simulink model "flightControlSystem"  (R2022a)
settings: Solver=ode3  StartTime=0  StopTime=TFinal  FixedStep=Ts  RelTol=1e-3  EnableMultiTasking=on
model workspace (MAT data in the model file):
  CIRCLE_PTS = [19 19 19]
  ZEROS = [0 0 0 0 0 0 0 0 0 0 0 0 ... (1444 elements, 38x38)]
undefined symbols (not defined in the file): codertarget, Controller, DiscIntNeverNeededParam, Discrete, Estimator, g, gray, init, orient_ref, pos_ref, Rec, SDTV, Sensors, Time, Ts, var_acc_angle_N, var_bias_gyr_N, var_gyro_p_N, Vehicle
libraries: simulink x38, visiontextngfix x7, visionconversions x5, slpidlib x4, ctrlSharedLib x4, sharedtransform x3, visionanalysis x1, parrotlib x1
(part 3 of 3)

== system flightControlSystem/Control System/State Estimator/XY Position Estimator/EstimatorVelocity/xy velocity w//o angular velocity compensation ==
  note: Optical flow raw readings are converted to velocity in m/s based on the estimated altitude
  optical_flow : Inport
  z_estimate : Inport  Port=2
  " " : Product  Inputs=**
  Compare To Constant : simulink/Logic and Bit Operations/Compare To Constant  relop=<  const=200*4  OutDataTypeStr=boolean
  Counter Free-Running : simulink/Sources/Counter Free-Running  NumBits=32  tsamp=-1
  Gain : Gain  Gain=-1
  Select dxy : Selector  InputPortWidth=3  IndexOptions=Index vector (dialog)  Indices=[1 2]  OutputSizes=1
  Switch : Switch  Criteria=u2 > Threshold  SaturateOnIntegerOverflow=off  InputSameDT=off
  opticalFlowErrorCorrect : Gain  Gain=1.15
  optical_flow_dx_dy : Outport
  wires:
  Select dxy/1 -> optical_flow_dx_dy/1  "optical_flow_dx_dy"
  " "/1 -> opticalFlowErrorCorrect/1
  opticalFlowErrorCorrect/1 -> Switch/3
  Gain/1 -> " "/2
  Switch/1 -> Select dxy/1
  Counter Free-Running/1 -> Compare To Constant/1
  Compare To Constant/1 -> Switch/2
  optical_flow/1 -> " "/1, Switch/1
  z_estimate/1 -> Gain/1

== matlab function flightControlSystem/Control System/Path Planning/way_parser ==
  data: x output; u input; y output; land output; r output; hough input; theta output
function [x, y, land,r, theta] = fcn(u,hough)

x = u(1);
y = u(2);
land = u(3);
r = hough(1);
theta = hough(2);

end

== matlab function flightControlSystem/Image Processing System/Bresenham Algorithm/circle_detection ==
  data: u input; detected output; shape input; way output
function [detected, way] = fcn(u, shape)

persistent landing;
if isempty(landing)
    landing = 0;
end

detected = 0;
way = [0 0 0];
land = 0;

if landing == 1
    way = [0 0 1];
    detected = 1;

else
    [total_pixel, cord_x, cord_y] = detect_circle(u, shape);
    
    if total_pixel >= 1350
        detected = 1;
        center_x = cord_x + 19;
        center_y = cord_y + 19;
    
        if center_x > 120
            center_x = 120;
        end
        if center_y > 160
            center_y = 160;
        end
        
        
        dif_x = round(60 - center_x);
        dif_y = round(center_y - 80);
        
        dist = sqrt(dif_x * dif_x + dif_y * dif_y);
    
        fprintf(' #### CIRCLE - centers: %3.1f %3.1f | dist: %3.1f\n', ...
            center_x, center_y, dist);
    
        if dist < 15
            land = 1;
            landing = 1;
        end
        way_x = dif_x / 130000;
        way_y = dif_y / 130000;
        way = [way_x way_y land];
    end

end

end

function [total_pixel, cord_x, cord_y] = detect_circle(u, shape)

%  total_pixel: sum of number of pixel
%       cord_x: row coordinate of u
%       cord_y: column coordinate of u

[circle_size_x, circle_size_y] = size(shape);
R = 120;  C = 160;

total_pixel = 0;
cord_x = 0;
cord_y = 0;

for i = 1:(R - circle_size_x)
    for j = 1:(C - circle_size_y)
        section = u(i:i+circle_size_x-1, j:j+circle_size_y-1);
        result = sum(~xor(section, shape), 'all');
        if result > total_pixel
            total_pixel = result;
            cord_x = i;
            cord_y = j;
        end
    end

end
end

== matlab function flightControlSystem/Image Processing System/Bresenham Algorithm/opposite_way ==
  data: way_x output; prev_xy input; way_y output
function [way_x, way_y] = fcn(prev_xy)

    x = prev_xy(1);
    y = prev_xy(2);
    
    if x == 0 || y == 0
        way_x = 0;
        way_y = 0;
    else
        way_x = 60 + (60 - x) + 1;
        way_y = 80 + (80 - y) + 1;
    end

    %fprintf('opposite: %.0f %.0f -> %.0f %.0f\n', x, y, way_x, way_y);
end

== matlab function flightControlSystem/Image Processing System/Hough Line Detecting/MATLAB Function4 ==
  data: bw input; cx output; cy output
function [cx, cy] = mid_point_of_line(bw)
%% FOR DEBUG
DEBUG = 0;
%%

[row,col] = find(bw);
n = length(row);

cx = 0;
cy = 0;
for ii = 1:n
    cx = cx + col(ii);
    cy = cy + row(ii);
end

cx = cx / n;
cy = cy / n;
if DEBUG == 1
    fprintf("cx = %f, cy = %f" , cx, cy);
end

== matlab function flightControlSystem/Image Processing System/Hough Line Detecting/MATLAB Function5 ==
  data: center_point input; r output; Ref_point input; theta output
%% r, that 구하는 함수
% Ref_point = [Line Edge 중점의 x 좌표, Line Edge 중점의 y 좌표]
% center_point = [ 드론 카메라의 기준점의 x, y 좌표] 
% 두개다 1차원 벡터 성분.
% 출력값: theta = [rad], r = 픽셀거리

function  [r, theta] =  calc_r_theta(center_point, Ref_point)
if(isreal(Ref_point))
    r = sqrt((Ref_point(1) - center_point(1))^2 + (Ref_point(2) - center_point(2))^2);
    theta = atan((Ref_point(2) - center_point(2)) / (Ref_point(1) - center_point(1)));
else
    r = 0;
    theta = 0;
end

== matlab function flightControlSystem/Image Processing System/Bresenham Algorithm/range_points ==
  data: x input; x1 output; y input; ref input; y1 output; x2 output; y2 output
function [x1,y1, x2,y2] = get_range_points(x,y, ref)

% x1, y1 are left
% x2, y2 are right 
% according to center-to-edge vector.

W = edge_number(x,y);

if W == 1
    y1 = y - ref;
    if y1 < 1
        x1 = x - y1;
        y1 = 1;
    else
        x1 = x;
    end

    y2 = y + ref;
    if y2 > 160
        x2 = y2-160;
        y2 = 160;
    else
        x2 = x;
    end
elseif W == 2
    x1 = x + ref;
    if x1 > 120
        y1 = x1 - 120;
        x1 = 120;
    else
        y1 = y;
    end

    x2 = x - ref;
    if x2 < 1
        y2 = abs(x2) + 1;
        x2 = 1;
    else
        y2 = y;
    end
elseif W == 4
    x1 = x - ref;
    if x1 < 1
        y1 = 160 + x1;
        x1 = 1;
    else
        y1 = 160;
    end

    x2 = x + ref;
    if x2 > 120
        y2 = 160 - (x2 - 120);
        x2 = 120;
    else
        y2 = y;
    end
elseif W == 3
    y1 = y + ref;
    if y1 > 160
        x1 = 120 - (y1-160);
        y1 = 160;
    else
        x1 = x;
    end

    y2 = y - ref;
    if y2 < 1
        x2 = 120 + y2;
        y2 = 1;
    else
        x2 = x;
    end
else
    x1 = 1; y1 = 1;
    x2 = 1; y2 = 2;
end

%fprintf('range_points: %.0f-%.0f  to  %.0f-%.0f\n', x1,y1, x2,y2);

end

== matlab function flightControlSystem/Image Processing System/Bresenham Algorithm/scan_range ==
  data: way output; u input; x1 input; y1 input; x2 input; y2 input; is_scan input
function way  = scan_range(u, x1,y1, x2,y2, is_scan)

way_x = 1;
way_y = 2;
speed = 0;
in_red_line = u(60, 80);


persistent prev_endless_x;
persistent prev_endless_y;

if is_scan
    if in_red_line == 1  % ------ inside red-line ------
    
        t = 0;
        mx = 0;

        mx_endless_x = [0 0];
        mx_endless_y = [0 0];
        mx_t = [0 0];

        last_endless = false;
        index_of_endless = 0;
        
        w1 = edge_number(x1,y1);
        xi = x1;  yi = y1; k = 1;
        
        if w1 == 1 || w1 == 4
            k = -1;
        end
        
        
        while xi ~= x2 || yi ~= y2
            returned = line_drawer(60, 80, xi, yi, u, 0);

            if returned == 0 % if endless

                if last_endless == false
                    last_endless = true;
                    index_of_endless = index_of_endless + 1;
                end
                if index_of_endless > 2
                    break;
                end
                
                mx_endless_x(index_of_endless) = mx_endless_x(index_of_endless) + xi;
                mx_endless_y(index_of_endless) = mx_endless_y(index_of_endless) + yi;
                mx_t(index_of_endless) = mx_t(index_of_endless) + 1;

            else
                last_endless = false;
                if returned > mx
                    mx = returned;
                    way_x = xi; 
                    way_y = yi;
                    t = 1;
                end
            end

            % İteration
            temp_w = edge_number(xi, yi);
            if temp_w == 1 || temp_w == 3
                yi = yi + k;
            else
                xi = xi + k;
            end
            if xi < 1
                yi = 159; xi = 1; k = -1;
            elseif xi > 120
                xi = 120; yi = 2; k = 1;
            elseif yi < 1
                yi = 1; xi = 2; k = 1;
            elseif yi > 160
                yi = 160; xi = 119; k = -1;
            end
        end % while end


        if index_of_endless == 1 % ---------- 1 endless ------------
            %fprintf('only one endless!\n');
            way_x = mx_endless_x(1);
            way_y = mx_endless_y(1);
            t = mx_t(1);

            way_x = round(way_x/t);
            way_y = round(way_y/t);
            [way_x, way_y] = nearest_edge(way_x, way_y);

            prev_endless_x = 60 + (60 - way_x) + 1;
            prev_endless_y = 80 + (80 - way_y) + 1;

        elseif index_of_endless == 2 % ---------- 2 endless ------------
            
            if isempty(prev_endless_x)
                way_x = mx_endless_x(1);
                way_y = mx_endless_y(1);
                t = mx_t(1);
    
                way_x = round(way_x/t);
                way_y = round(way_y/t);
                [way_x, way_y] = nearest_edge(way_x, way_y);
    
                prev_endless_x = 60 + (60 - way_x) + 1;
                prev_endless_y = 80 + (80 - way_y) + 1;
            else
                mid_calculated = [0 0; 0 0];
                for i = 1:2
                    x = mx_endless_x(i);
                    y = mx_endless_y(i);
                    t = mx_t(i);

                    x = round(x/t);
                    y = round(y/t);
                    
                    [x,y] = nearest_edge(x, y);
                    
                    mid_calculated(i, 1) = x;
                    mid_calculated(i, 2) = y;
                end
                %fprintf('calculated = %.0f %.0f  | %.0f %.0f\n', ...
                %    mid_calculated(1,1), mid_calculated(1,2), ...
                %    mid_calculated(2,1), mid_calculated(2,2));

                diff_x1 = prev_endless_x-mid_calculated(1,1);
                diff_y1 = prev_endless_y-mid_calculated(1,2);
                diff_x2 = prev_endless_x-mid_calculated(2,1);
                diff_y2 = prev_endless_y-mid_calculated(2,2);
                diff1 = sqrt(diff_x1*diff_x1 + diff_y1*diff_y1);
                diff2 = sqrt(diff_x2*diff_x2 + diff_y2*diff_y2);

                if diff1 > diff2
                    way_x = mid_calculated(1,1);
                    way_y = mid_calculated(1,2);
                else
                    way_x = mid_calculated(2,1);
                    way_y = mid_calculated(2,2);
                end
                
                prev_endless_x = 60 + (60 - way_x) + 1;
                prev_endless_y = 80 + (80 - way_y) + 1;
                
            end
        else % ---------- NO endless ------------
            speed = mx;
        end

        

    else % ----------------- outside red line ----------------------
        x1 = 2; y1 = 1;
        x2 = 1; y2 = 1;
        
        ENDLESS = 100;
        mn = ENDLESS;
        w1 = edge_number(x1,y1);
        xi = x1;  yi = y1;  k = 1;
        if w1 == 1 || w1 == 4
            k = -1;
        end
        
        while xi ~= x2 || yi ~= y2
            returned = line_drawer(60, 80, xi, yi, u, 1);
    
            if returned > 0 && returned < mn
                mn = returned;
                way_x = xi;
                way_y = yi;
            end
    
            % İteration
            temp_w = edge_number(xi, yi);
            if temp_w == 1 || temp_w == 3
                yi = yi + k;
            else
                xi = xi + k;
            end
            if xi < 1
                yi = 159; xi = 1; k = -1;
            elseif xi > 120
                xi = 120; yi = 2; k = 1;
            elseif yi < 1
                yi = 1; xi = 2; k = 1;
            elseif yi > 160
                yi = 160; xi = 119; k = -1;
            end
        end % while
        
        speed = 100;
        if mn < 60
            speed = 60;
        end
    end % if redline end

end % is_scan

way = [way_x, way_y, speed];

end % function end

== matlab function flightControlSystem/Image Processing System/Bresenham Algorithm/speed_calculator ==
  data: way input; X output; Y output
function [X,Y] = fcn(way)

x = way(1);
y = way(2);
speed = way(3);

if speed == 100
    speed = 200;
elseif speed < 60
    speed = 60;
end


X = (60-x) / 10000000 * speed;
Y = (y-80) / 10000000 * speed;


%fprintf(' --- speed: %f | ', speed); fprintf('vectors: X=%.5f | Y=%.5f\n', X, Y);

end

== matlab function flightControlSystem/Image Processing System/Bresenham Algorithm/visualize_helper ==
  data: r input; R output; g input; b input; way_x input; way_y input; G output; B output; lx input; ly input; rx input; ry input
function [R,G,B] = fcn(r,g,b, way_x, way_y,  lx,ly, rx,ry)

% completely unnecessary block for algorithm, just for visualize

r(60,80) = 255; g(60,80) = 255; b(60,80) = 255;

if way_x >= 1 && way_y >= 1 && way_x <= 120 && way_y <= 160


% -----------------------------------------------
    x1 = 60; y1 = 80;  x2 = way_x;   y2 = way_y;
    swapepd = 0;
    if abs(y2 - y1) > abs(x2 - x1)
        %disp('[swapped] dy bigger')
        swapepd = 1;
        [x1,y1] = deal(y1,x1);
        [x2,y2] = deal(y2,x2);
        xk = 1; yk = 1;
        if (x2 < x1) xk = -1; end
        if (y2 < y1) yk = -1; end
    else
        xk = -1; yk = -1;
        if (x2 > x1) xk = 1; end
        if (y2 > y1) yk = 1; end

    end
    dy = abs(y2-y1);
    dx = abs(x2-x1);
    % --------------------------------------
    m = 2 * dy;
    slope_error = m - 2*dx;
  
    y = y1;
    for x = x1:xk:x2
        if swapepd == 1
            r(y,x) = 255; g(y,x) = 255; b(y,x) = 255;
        else
            r(x,y) = 255; g(x,y) = 255; b(x,y) = 255;
        end
        
   
        slope_error = slope_error + m;
        if (slope_error > 0)
            y = y + yk;
            slope_error = slope_error - 2 * dx;
        end
    end
end




% --------------------------------------------
x1 = 60; y1 = 80; x2 = lx; y2 = ly;
    swapepd = 0;
    if abs(y2 - y1) > abs(x2 - x1)
        %disp('[swapped] dy bigger')
        swapepd = 1;
        [x1,y1] = deal(y1,x1);
        [x2,y2] = deal(y2,x2);
        xk = 1; yk = 1;
        if (x2 < x1) xk = -1; end
        if (y2 < y1) yk = -1; end
    else
        xk = -1; yk = -1;
        if (x2 > x1) xk = 1; end
        if (y2 > y1) yk = 1; end

    end
    dy = abs(y2-y1);
    dx = abs(x2-x1);
    % --------------------------------------
    m = 2 * dy;
    slope_error = m - 2*dx;
  
    y = y1;
    for x = x1:xk:x2
        if swapepd == 1
            g(y,x) = 255;
        else
            g(x,y) = 255;
        end
        
   
        slope_error = slope_error + m;
        if (slope_error > 0)
            y = y + yk;
            slope_error = slope_error - 2 * dx;
        end
    end
% -----------------------------------------

    x1 = 60; y1 = 80; x2 = rx; y2 = ry;
    swapepd = 0;
    if abs(y2 - y1) >= abs(x2 - x1)
        %disp('[swapped] dy bigger')
        swapepd = 1;
        [x1,y1] = deal(y1,x1);
        [x2,y2] = deal(y2,x2);
        xk = 1; yk = 1;
        if (x2 < x1) xk = -1; end
        if (y2 < y1) yk = -1; end
    else
        xk = -1; yk = -1;
        if (x2 > x1) xk = 1; end
        if (y2 > y1) yk = 1; end

    end
    dy = abs(y2-y1);
    dx = abs(x2-x1);
    % --------------------------------------
    m = 2 * dy;
    slope_error = m - 2*dx;
  
    y = y1;
    for x = x1:xk:x2
        if swapepd == 1
            if x <1 break; end
            g(y,x) = 255;
        else
            g(x,y) = 255;
        end
        
   
        slope_error = slope_error + m;
        if (slope_error > 0)
            y = y + yk;
            slope_error = slope_error - 2 * dx;
        end
    end

b(40:80, 60:90) = 200;
R = r;
G = g;
B = b;
end

== matlab function flightControlSystem/Image Processing System/Bresenham Algorithm/write_or_not ==
  data: way input; way_out output; in_red input; prev_xy input; way_x output; way_y output
function [way_out, way_x, way_y] = fcn(way, in_red, prev_xy)

x = way(1);
y = way(2);
speed = way(3);

if in_red
    X = x;   Y = y;
    way_x = x;  way_y = y;
else
    X = x;  Y = y; 
    way_x = prev_xy(1);  
    way_y = prev_xy(2);
end

way_out = [X Y speed];

%fprintf('X = %f | Y = %f\n', way_x, way_y);
end

== matlab function flightControlSystem/Image Processing System/Bresenham Algorithm/center_vector_x ==
  data: u input; slide_x output
function slide_x = fcn(u)
c1 = 60; 
c2 = 80;
left_p = 0;
right_p = 0;
middle_point = u(c1, c2);
compare = ~middle_point;
for i = c2:-1:60 % <---  look left
    if u(c1, i) == compare
        left_p = i;
        break
    end
end
for i = c2:100 % --->   look right
    if u(c1, i) == compare
        right_p = i;
        break
    end
end

slide_x = 0;
if left_p ~= 0 && right_p ~= 0 % in line
    if middle_point == 1
        vr = right_p - c2;  % length right 
        vl = c2 - left_p;   % length left
        diff = vr-vl;
        slide_x = get_speed(diff) * 20;
    end
end
end

function T = get_speed(t)

if t > 0
    if t < 1
        T = 0.000001;
    elseif t < 5
        T = 0.000002;
    elseif t < 10
        T = 0.000003;
    elseif t < 15
        T = 0.000004;
    elseif t < 20
        T = 0.000005;
    else
        T = 0.000006;
    end
else
    if t < -20
        T = -0.000006;
    elseif t < -15
        T = -0.000005;
    elseif t < -10
        T = -0.000004;
    elseif t < -5
        T = -0.000003;
    elseif t < -1
        T = -0.000002;
    else
        T = -0.000001;
    end
end

end

== matlab function flightControlSystem/Control System/Controller/Position Controller/Position error transformation (Earth to Body frame) ==
  data: yaw input; xy_err_earth input; xy_err_body output
function xy_err_body = fcn(yaw,xy_err_earth)

transformation = [cos(yaw), sin(yaw); -sin(yaw),  cos(yaw)];
xy_err_body = transformation * xy_err_earth;


end

== matlab function flightControlSystem/Image Processing System/Bresenham Algorithm/center_vector_y ==
  data: u input; slide_y output
function slide_y = fcn(u)
c1 = 60; 
c2 = 80;
up_p = 0;
down_p = 0;
middle_point = u(c1,c2);
compare = ~middle_point;
for i = c1:-1:40 % look up
    if u(i, c2) == compare
        up_p = i;
        break
    end
end
for i = c1:80 % look down
    if u(i, c2) == compare
        down_p = i;
        break
    end
end
slide_y = 0;
if up_p ~= 0 && down_p ~= 0  % in line
    if middle_point == 1
        vu = down_p - c1;  %length up
        vd = c1 - up_p;    %length down
        diff = vd-vu;
        
        slide_y = get_speed(diff) * 20;
    end
end

end
function T = get_speed(t)

if t > 0
    if t <= 1
        T = 0.000001;
    elseif t < 5
        T = 0.000002;
    elseif t < 10
        T = 0.000003;
    elseif t < 15
        T = 0.000005;
    elseif t < 20
        T = 0.000005;
    else
        T = 0.000005;
    end
else
    if t < -20
        T = -0.000005;
    elseif t < -15
        T = -0.000005;
    elseif t < -10
        T = -0.000004;
    elseif t <= -5
        T = -0.000003;
    elseif t < -1
        T = -0.000002;
    else
        T = -0.000001;
    end
end
end

== matlab function flightControlSystem/Image Processing System/Hough Line Detecting/MATLAB Function ==
  data: u input; img_H output; img_S output; img_V output
function [img_H, img_S, img_V] = fcn(u)

img_H = u(:,:,1);
img_S = u(:,:,2);
img_V = u(:,:,3);

== matlab function flightControlSystem/Image Processing System/Bresenham Algorithm/check_last_way ==
  data: u input; is_scan output; in_red output; prev_xy input; DISTANCE input; way output
function [is_scan, in_red, way]  = fcn(u, prev_xy, DISTANCE)

prev_x = prev_xy(1);
prev_y = prev_xy(2);

in_red = u(60, 80);
compare = ~in_red;

is_scan = 0;
way_x = 1;
way_y = 1;
speed = 0;

if prev_x == 0 || prev_y == 0
    is_scan = 1;
else 
    if u(prev_x, prev_y) == 1 

        % endless continue ------------------------------
        [ref_x, ref_y] = middle_point_of_endless_line(u, prev_x, prev_y);

        way_x = prev_x + ref_x;
        way_y = prev_y + ref_y;
        
        if way_y > 160
            if way_x == 120 
                way_x = 120 - mod(way_y, 160);
            elseif way_x == 1 
                way_x = mod(way_y, 160);
            end
            way_y = 160;
            
        elseif way_y < 1
            if way_x == 120 
                way_x = 120 - abs(way_y);
            elseif way_x == 1 
                way_x = abs(way_y); 
            end
            way_y = 1;
            
        elseif way_x < 1
            if way_y == 160
                way_y = 160 - abs(way_x);
            elseif way_y == 1
                way_y = abs(way_x);
            end
            way_x = 1;
            
        elseif way_x > 120
            if way_y == 160
                way_y = 160 - (way_x - 120);
            elseif way_y == 1
                way_y = way_x - 120;
            end
            way_x = 120;
        end

        %{
        if way_x < 1   way_x = 1;   end
        if way_x > 120 way_x = 120; end
        if way_y < 1   way_y = 1;   end
        if way_y > 160 way_y = 160; end
        %}
        speed = 100;

    else 
        
        % endless dissappeared ----------------------------
        if in_red
            distance = line_drawer(60, 80, prev_x, prev_y, u, compare);
            if distance < DISTANCE
                is_scan = 1;
                speed = 0;
            else
                speed = distance;
            end
            
            way_x = prev_x;
            way_y = prev_y;
        else
            is_scan = 1;
            way_x = prev_x;
            way_y = prev_y;
            speed = 40;
        end

    end
end
way = [way_x, way_y, speed];

end % func end



function [ref_x, ref_y] = middle_point_of_endless_line(u, way_x, way_y)

w = edge_number(way_x, way_y);

if w == 1 || w == 3

    % to right
    iter_y = way_y;
    iter_x = way_x;
    plus_or_minus = 1;
    x_or_y = 0; % 0:y   1:x
    distance = 0;

    while u(iter_x, iter_y) == 1
        if x_or_y == 0
            iter_y = iter_y + plus_or_minus;
        else
            iter_x = iter_x + plus_or_minus;
        end
        distance = distance + 1;
        
        if iter_y > 160
            iter_y = 160;
            x_or_y = 1;
            if iter_x == 120
                plus_or_minus = -1;
            elseif iter_x == 1
                plus_or_minus = 1;
            end
        end
        if iter_x < 1
            break;
        elseif iter_x > 120
            break;
        end
    end
    right = distance;

    % to left
    iter_y = way_y;
    iter_x = way_x;
    plus_or_minus = -1;
    x_or_y = 0; % 0:y   1:x
    distance = 0;
    
    while u(iter_x, iter_y) == 1
        if x_or_y == 0
            iter_y = iter_y + plus_or_minus;
        else
            iter_x = iter_x + plus_or_minus;
        end
        distance = distance + 1;

        if iter_y < 1
            iter_y = 1;
            x_or_y = 1;
            if iter_x == 120
                plus_or_minus = -1;
            elseif iter_x == 1
                plus_or_minus = 1;
            end
        end
        if iter_x < 1
            break
        elseif iter_x > 120
            break
        end
    end
    left = distance;
    
    
    ref_x = 0;
    diff = right - left;
    
    if abs(diff) >= 7 && abs(diff) < 25
        ref_y = round(diff/2);
    else
        ref_y = 0;
    end

else % ------------------------- 2 & 4 --------------------------
    % to up
    iter_x = way_x;
    iter_y = way_y;
    plus_or_minus = -1;
    x_or_y = 1; % 0:y   1:x
    distance = 0;
    while u(iter_x, iter_y) == 1
        if x_or_y == 0
            iter_y = iter_y + plus_or_minus;
        else
            iter_x = iter_x + plus_or_minus;
        end
        distance = distance + 1;

        if iter_x < 1
            iter_x = 1;
            x_or_y = 0;
            if iter_y == 1
                plus_or_minus = 1;
            elseif iter_y == 160
                plus_or_minus = -1;
            end
        end
        if iter_y > 160
            break
        elseif iter_y < 1
            break
        end
    end
    up = distance;

    % to down
    iter_x = way_x;
    iter_y = way_y;
    plus_or_minus = 1;
    x_or_y = 1; % 0:y   1:x
    distance = 0;
    while u(iter_x, iter_y) == 1
        if x_or_y == 0
            iter_y = iter_y + plus_or_minus;
        else
            iter_x = iter_x + plus_or_minus;
        end
        distance = distance + 1;
        if iter_x > 120
            x_or_y = 0;
            iter_x = 120;
            if iter_y == 1
                plus_or_minus = 1;
            elseif iter_y == 160
                plus_or_minus = -1;
            end
        end
        if iter_y > 160
            break;
        elseif iter_y < 1
            break;
        end
    end
    down = distance;

    diff = down - up;

    ref_y = 0;
    if abs(diff) >= 7 && abs(diff) < 25
        ref_x = round(diff/2);
    else
        ref_x = 0;
    end
end

end

== matlab function flightControlSystem/Image Processing System/Hough Line Detecting/MATLAB Function1 ==
  data: binary input; slope output; intercept output; cropImg output
function [slope, intercept,cropImg] = find_slope_intercept_from_binary(binary)
% FOR DEBUG
DEBUG = 1;
% 
cropImg = binary(60:120,65:95);  
[Lrows, Lcols] = find(cropImg);


n = length(Lrows);

if n > 500
    p = round(n/10);
    idx = randperm(n,p);

    x = Lrows(idx);
    y = Lcols(idx);

    p = polyfit(x,y,1);
    slope = p(1);
    intercept = p(2);

    if DEBUG == 1
    fprintf("find_slope_intercept_from_binary: slope = %8.4f , intercept = %8.4f", slope, intercept)
    end

else
    if DEBUG == 1
    disp("find_slope_intercept_from_binary: n is under 50 !")
    end

    slope = 0;
    intercept = 0;
end

== matlab function flightControlSystem/Image Processing System/Hough Line Detecting/MATLAB Function2 ==
  data: slope input; pts output; intercept input
function pts = slope_intercept_to_pts(slope, intercept)

x1 = 80;
y1 = 60;

theta = atan(slope);
r = 10;

x2 = x1 + r*cos(theta);
y2 = y1 + r*sin(theta);

pts = [x1, y1, x2, y2];

== matlab function flightControlSystem/Image Processing System/Hough Line Detecting/MATLAB Function3 ==
  data: bw input; bwmorph_img output
function bwmorph_img = fcn(bw)

bwmorph_img = bwmorph(bw,'skel', Inf);

== stateflow chart flightControlSystem/Control System/Path Planning/Chart ==
  state hover
    xout = 0;
    yout = 0;
    zout = -1.5;
  state go
    xout = xout+0.001*cos(yaw);
    yout = yout+0.001*sin(yaw);
    zout = -1.5;
  state land
    zout = zout + 0.004;
    xout = xout;
    yout = yout;
  state Yawing
    if theta < 0
    yaw = yaw + 0.0005;
    else
    yaw = yaw - 0.0005;
    end
  (default) -> hover
  go -> land [order 1] : [land == 1]
  Yawing -> go : [abs(abs(theta)-1.5) < 0.1]
  hover -> Yawing : after(3,sec)
  go -> Yawing [order 2] : [abs(abs(theta)-1.5) > 0.1]
  data: xout output; yout output; zout output; land input; theta input; yaw output =0
